simulink model "PCM_Decoder"  (R2021a)
settings: Solver=VariableStepAuto  StartTime=0.0  StopTime=2e-3  FixedStep=1/(48e-7)  MaxStep=1e-5  RelTol=1e-3
model workspace (MAT data in the model file):
  adcLowerSaturation = -2.5
  adcUpperSaturation = 2.5
  decimationFactor = 3
  samplingFrequency = 48000
  transmissionBitDepth = 4
  transmissionFrequency = 16000
values from neighbouring files (symbols this model uses):
  hzDen = [1 zeros(1,(length(hzNum)-1))]    [FIRMaker.m]
  hzNum = zeros(1,tap)    [FIRMaker.m]
libraries: simulink x8, dspquant2 x1, dspsigops x1
settings Model: OrderedModelArguments=off  Creator=james  LastModifiedBy=james

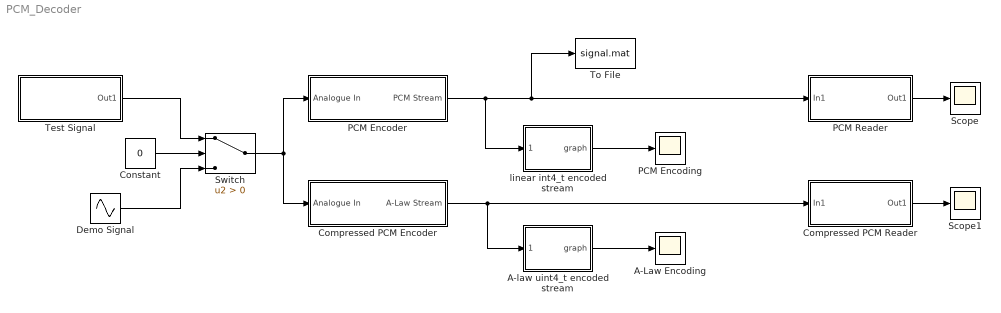
== system PCM_Decoder ==
  A-Law Encoding : Scope
  A-law uint4_t encoded stream : Subsystem
  Compressed PCM Encoder : Subsystem
  Compressed PCM Reader : Subsystem
  Constant : Constant  Value=0
  Demo Signal : Sin  Amplitude=2.4  Frequency=4000  SampleTime=0
  PCM Encoder : Subsystem
  PCM Encoding : Scope
  PCM Reader : Subsystem
  Scope : Scope
  Scope1 : Scope
  Switch : Switch  Criteria=u2 > Threshold
  Test Signal : Subsystem
  To File : ToFile  Filename=signal.mat  SaveFormat=Timeseries
  linear int4_t encoded stream : Subsystem
  wires:
  PCM Encoder/1(PCM Stream) -> To File/1, PCM Reader/1(In1), linear int4_t encoded stream/1(uint4_t)
  linear int4_t encoded stream/1(graph) -> PCM Encoding/1
  A-law uint4_t encoded stream/1(graph) -> A-Law Encoding/1
  Constant/1 -> Switch/2
  Switch/1 -> Compressed PCM Encoder/1(Analogue In), PCM Encoder/1(Analogue In)
  Compressed PCM Encoder/1(A-Law Stream) -> A-law uint4_t encoded stream/1(uint4_t), Compressed PCM Reader/1(In1)
  Test Signal/1(Out1) -> Switch/1
  Demo Signal/1 -> Switch/3
  PCM Reader/1(Out1) -> Scope/1
  Compressed PCM Reader/1(Out1) -> Scope1/1

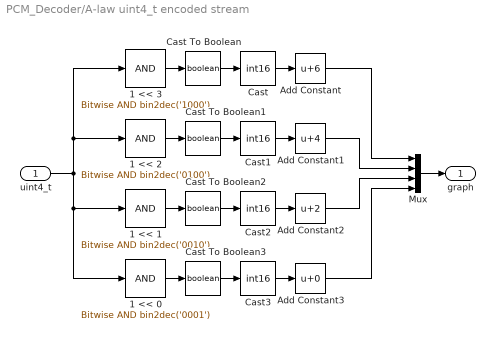
== system PCM_Decoder/A-law uint4_t encoded stream ==
  uint4_t : Inport
  1 << 0 : simulink/Logic and Bit Operations/Bitwise Operator  logicop=AND  UseBitMask=on  BitMask=bin2dec('0001')  BitMaskRealWorld=Stored Integer
  1 << 1 : simulink/Logic and Bit Operations/Bitwise Operator  logicop=AND  UseBitMask=on  BitMask=bin2dec('0010')  BitMaskRealWorld=Stored Integer
  1 << 2 : simulink/Logic and Bit Operations/Bitwise Operator  logicop=AND  UseBitMask=on  BitMask=bin2dec('0100')  BitMaskRealWorld=Stored Integer
  1 << 3 : simulink/Logic and Bit Operations/Bitwise Operator  logicop=AND  UseBitMask=on  BitMask=bin2dec('1000')  BitMaskRealWorld=Stored Integer
  Add Constant : Bias  Bias=6
  Add Constant1 : Bias  Bias=4
  Add Constant2 : Bias  Bias=2
  Add Constant3 : Bias
  Cast{,1..3} (4 alike) : DataTypeConversion  OutDataTypeStr=int16
  Cast To Boolean{,1..3} (4 alike) : DataTypeConversion  OutDataTypeStr=boolean
  Mux : Mux
  graph : Outport
  wires:
  uint4_t/1 -> 1 << 0/1, 1 << 1/1, 1 << 3/1, 1 << 2/1
  Mux/1 -> graph/1
  1 << 2/1 -> Cast To Boolean1/1
  1 << 1/1 -> Cast To Boolean2/1
  1 << 0/1 -> Cast To Boolean3/1
  1 << 3/1 -> Cast To Boolean/1
  Cast To Boolean/1 -> Cast/1
  Cast/1 -> Add Constant/1
  Add Constant/1 -> Mux/1
  Add Constant1/1 -> Mux/2
  Cast1/1 -> Add Constant1/1
  Cast To Boolean1/1 -> Cast1/1
  Add Constant2/1 -> Mux/3
  Cast To Boolean2/1 -> Cast2/1
  Cast2/1 -> Add Constant2/1
  Cast3/1 -> Add Constant3/1
  Add Constant3/1 -> Mux/4
  Cast To Boolean3/1 -> Cast3/1

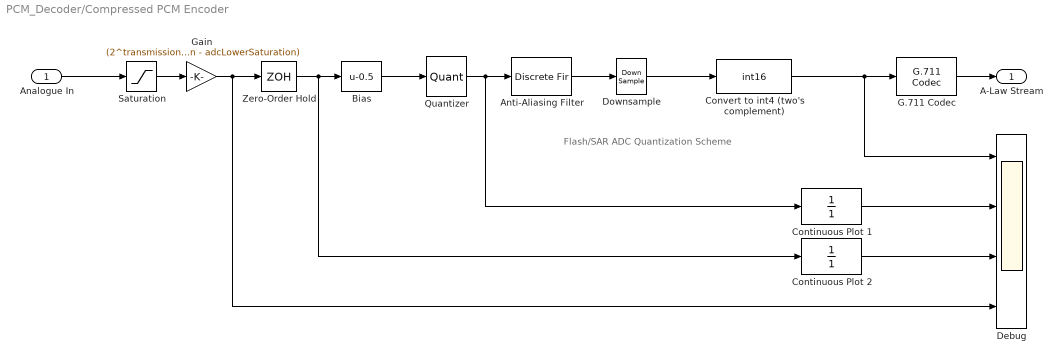
== system PCM_Decoder/Compressed PCM Encoder ==
  note: Flash/SAR ADC Quantization Scheme
  Analogue In : Inport
  Anti-Aliasing Filter : DiscreteFir
  Bias : Bias  Bias=-0.5
  Continuous Plot 1 : TransferFcn  Denominator=[1]  ContinuousStateAttributes="''Continuous\""
  Continuous Plot 2 : TransferFcn  Denominator=[1]  ContinuousStateAttributes="''Continuous\""
  Convert to int4 (two's complement) : DataTypeConversion  OutDataTypeStr=int16
  Debug : Scope  NumInputPorts=4
  Downsample : DownSample  N=3  RateOptions=Allow multirate processing
  G.711 Codec : dspquant2/G.711 Codec  mode=Encode PCM to A-law  errmode=Warning
      settings: SourceProductBaseCode=DS
  Gain : Gain  Gain=(2^transmissionBitDepth - 1)/(adcUpperSaturation - adcLowerSaturation)
  Quantizer : Quantizer  QuantizationInterval=1  LinearizeAsGain=off
  Saturation : Saturate  UpperLimit=2.5  LowerLimit=-2.5
  Zero-Order Hold : ZeroOrderHold  SampleTime=1/samplingFrequency
  A-Law Stream : Outport
  wires:
  Saturation/1 -> Gain/1
  Gain/1 -> Debug/4, Zero-Order Hold/1
  Bias/1 -> Quantizer/1
  Convert to int4 (two's complement)/1 -> Debug/1, G.711 Codec/1
  Zero-Order Hold/1 -> Bias/1, Continuous Plot 2/1
  Downsample/1 -> Convert to int4 (two's complement)/1
  Anti-Aliasing Filter/1 -> Downsample/1
  Quantizer/1 -> Continuous Plot 1/1, Anti-Aliasing Filter/1
  Continuous Plot 1/1 -> Debug/2
  Continuous Plot 2/1 -> Debug/3
  Analogue In/1 -> Saturation/1
  G.711 Codec/1 -> A-Law Stream/1

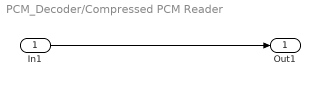
== system PCM_Decoder/Compressed PCM Reader ==
  In1 : Inport
  Out1 : Outport
  wires:
  In1/1 -> Out1/1

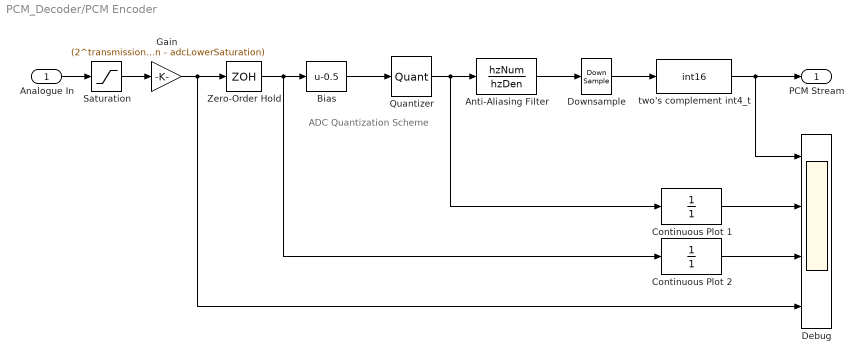
== system PCM_Decoder/PCM Encoder ==
  note: ADC Quantization Scheme
  Analogue In : Inport
  Anti-Aliasing Filter : DiscreteTransferFcn  Numerator=hzNum  Denominator=hzDen
  Bias : Bias  Bias=-0.5
  Continuous Plot 1 : TransferFcn  Denominator=[1]  ContinuousStateAttributes="''Continuous\""
  Continuous Plot 2 : TransferFcn  Denominator=[1]  ContinuousStateAttributes="''Continuous\""
  Debug : Scope  NumInputPorts=4
  Downsample : DownSample  N=decimationFactor  RateOptions=Allow multirate processing
  Gain : Gain  Gain=(2^transmissionBitDepth - 1)/(adcUpperSaturation - adcLowerSaturation)
  Quantizer : Quantizer  QuantizationInterval=1  LinearizeAsGain=off
  Saturation : Saturate  UpperLimit=2.5  LowerLimit=-2.5
  Zero-Order Hold : ZeroOrderHold  SampleTime=1/samplingFrequency
  two's complement int4_t : DataTypeConversion  OutDataTypeStr=int16
  PCM Stream : Outport
  wires:
  Saturation/1 -> Gain/1
  Gain/1 -> Debug/4, Zero-Order Hold/1
  Bias/1 -> Quantizer/1
  two's complement int4_t/1 -> PCM Stream/1, Debug/1
  Zero-Order Hold/1 -> Bias/1, Continuous Plot 2/1
  Downsample/1 -> two's complement int4_t/1
  Anti-Aliasing Filter/1 -> Downsample/1
  Quantizer/1 -> Anti-Aliasing Filter/1, Continuous Plot 1/1
  Continuous Plot 1/1 -> Debug/2
  Continuous Plot 2/1 -> Debug/3
  Analogue In/1 -> Saturation/1

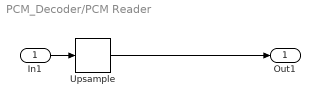
== system PCM_Decoder/PCM Reader ==
  In1 : Inport
  Upsample : dspsigops/Upsample  N=decimationFactor  phase=0  RateOptions=Allow multirate processing  ic=0  mode=Unused parameter value
  Out1 : Outport
  wires:
  In1/1 -> Upsample/1
  Upsample/1 -> Out1/1

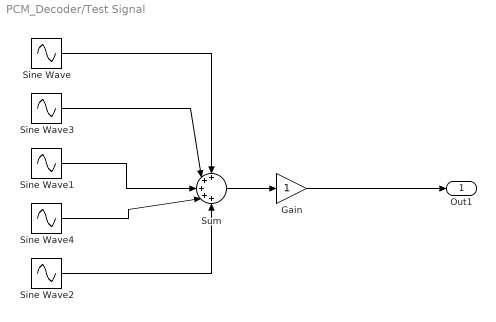
== system PCM_Decoder/Test Signal ==
  Gain : Gain
  Sine Wave : Sin  Frequency=677  SampleTime=0
  Sine Wave1 : Sin  Frequency=550  SampleTime=0
  Sine Wave2 : Sin  Frequency=6500  SampleTime=0
  Sine Wave3 : Sin  Frequency=4200  SampleTime=0
  Sine Wave4 : Sin  Frequency=1200  SampleTime=0
  Sum : Sum  Inputs=+++++
  Out1 : Outport
  wires:
  Sine Wave1/1 -> Sum/3
  Gain/1 -> Out1/1
  Sine Wave3/1 -> Sum/2
  Sine Wave/1 -> Sum/1
  Sum/1 -> Gain/1
  Sine Wave4/1 -> Sum/4
  Sine Wave2/1 -> Sum/5

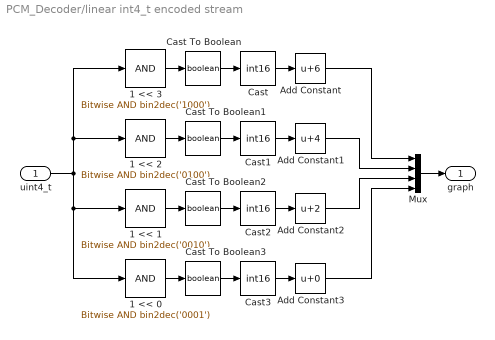
== system PCM_Decoder/linear int4_t encoded stream ==
  uint4_t : Inport
  1 << 0 : simulink/Logic and Bit Operations/Bitwise Operator  logicop=AND  UseBitMask=on  BitMask=bin2dec('0001')  BitMaskRealWorld=Stored Integer
  1 << 1 : simulink/Logic and Bit Operations/Bitwise Operator  logicop=AND  UseBitMask=on  BitMask=bin2dec('0010')  BitMaskRealWorld=Stored Integer
  1 << 2 : simulink/Logic and Bit Operations/Bitwise Operator  logicop=AND  UseBitMask=on  BitMask=bin2dec('0100')  BitMaskRealWorld=Stored Integer
  1 << 3 : simulink/Logic and Bit Operations/Bitwise Operator  logicop=AND  UseBitMask=on  BitMask=bin2dec('1000')  BitMaskRealWorld=Stored Integer
  Add Constant : Bias  Bias=6
  Add Constant1 : Bias  Bias=4
  Add Constant2 : Bias  Bias=2
  Add Constant3 : Bias
  Cast{,1..3} (4 alike) : DataTypeConversion  OutDataTypeStr=int16
  Cast To Boolean{,1..3} (4 alike) : DataTypeConversion  OutDataTypeStr=boolean
  Mux : Mux
  graph : Outport
  wires:
  uint4_t/1 -> 1 << 0/1, 1 << 1/1, 1 << 3/1, 1 << 2/1
  Mux/1 -> graph/1
  1 << 2/1 -> Cast To Boolean1/1
  1 << 1/1 -> Cast To Boolean2/1
  1 << 0/1 -> Cast To Boolean3/1
  1 << 3/1 -> Cast To Boolean/1
  Cast To Boolean/1 -> Cast/1
  Cast/1 -> Add Constant/1
  Add Constant/1 -> Mux/1
  Add Constant1/1 -> Mux/2
  Cast1/1 -> Add Constant1/1
  Cast To Boolean1/1 -> Cast1/1
  Add Constant2/1 -> Mux/3
  Cast To Boolean2/1 -> Cast2/1
  Cast2/1 -> Add Constant2/1
  Cast3/1 -> Add Constant3/1
  Add Constant3/1 -> Mux/4
  Cast To Boolean3/1 -> Cast3/1
